simulink model "Circuito"  (R2016b)
settings: Solver=VariableStepAuto  StartTime=0  StopTime=3e-3  RelTol=1e-3
libraries: powerlib x15
settings Model: Creator=Usuario  LastModifiedBy=Usuario
settings DataIOCC: LoggingIntervals=[2e-3, 3e-3]

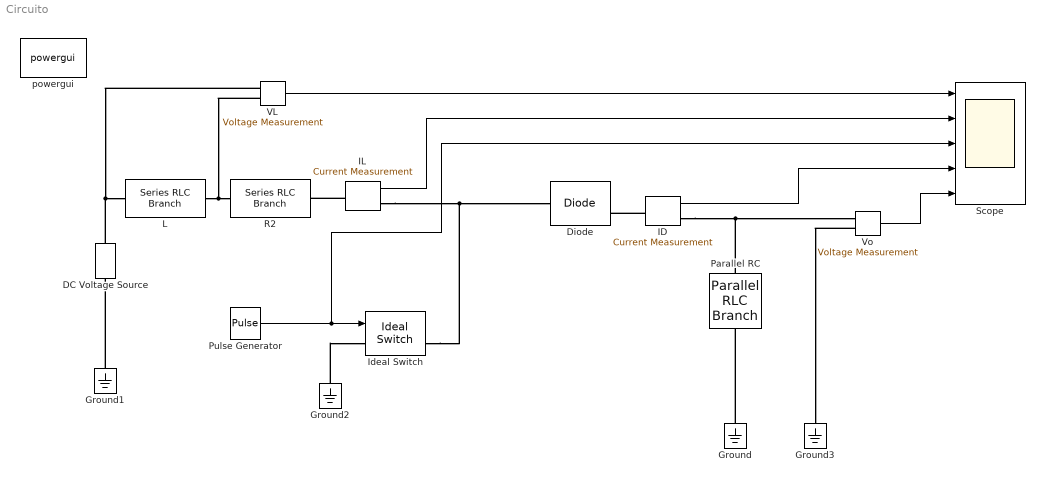
== system Circuito ==
  DC Voltage Source : powerlib/Electrical Sources/DC Voltage Source  Amplitude=12  Measurements=None
  Diode : powerlib/Power Electronics/Diode  Ron=0.001  Lon=0  Vf=0.8  IC=0  UseSnubber=off  Rs=500  Cs=250e-9  Measurements=on
  Ground{,1..3} (4 alike) : powerlib/Elements/Ground  LConnTagsString=a
  ID : powerlib/Measurements/Current Measurement  PhasorSimulation=off  OutputType=Complex  PSBequivalent=0
  IL : powerlib/Measurements/Current Measurement  PhasorSimulation=off  OutputType=Complex  PSBequivalent=0
  Ideal Switch : powerlib/Power Electronics/Ideal Switch  Ron=0.001  Lon=0  IC=0  Rs=1e5  Cs=inf  Measurements=on
  L : powerlib/Elements/Series RLC Branch  LConnTagsString=__new0  RConnTagsString=__new0  BranchType=L  Resistance=1  Inductance=220e-6  SetiL0=off  InitialCurrent=0  Capacitance=1e-6  Setx0=off  InitialVoltage=0  Measurements=None
  Parallel RC : powerlib/Elements/Parallel RLC Branch  LConnTagsString=a  RConnTagsString=__new0  BranchType=RC  Resistance=100  Inductance=0  SetiL0=off  InitialCurrent=0  Capacitance=10e-6  Setx0=off  InitialVoltage=0  Measurements=None
  Pulse Generator : DiscretePulseGenerator  PulseType=Time based  Period=16.667e-6  PulseWidth=54.38447187
  R2 : powerlib/Elements/Series RLC Branch  LConnTagsString=__new0  RConnTagsString=__new0  BranchType=R  Resistance=2  Inductance=1e-3  SetiL0=off  InitialCurrent=0  Capacitance=1e-6  Setx0=off  InitialVoltage=0  Measurements=None
  Scope : Scope  NumInputPorts=5
  VL : powerlib/Measurements/Voltage Measurement  PhasorSimulation=off  OutputType=Complex  PSBequivalent=0
  Vo : powerlib/Measurements/Voltage Measurement  PhasorSimulation=off  OutputType=Complex  PSBequivalent=0
  powergui : powerlib/powergui  Priority=1  SimulationMode=Continuous  SolverType=Tustin/Backward Euler (TBE)  SampleTime=50e-6  frequency=60  SPID=on  DisableSnubberDevices=off  DisableRonSwitches=off  DisableVfSwitches=off  SwTol=0  DisplayEquations=off  Interpol=off  ExternalGateDelay=off  methode=off  Ts=10  FunctionMessages=off  echomessages=off  HookPort=off  EnableUseOfTLC=off  x0status=blocks  frequencyindice=0  Pbase=100e6  ErrMax=1e-4  Iterations=50  UnitsV=kV  UnitsW=MW  buscounter=0  RestoreLinks=warning  ResistiveCurrentMeasurement=off  Frange=[0:2:500]  Ylog=off  Xlog=on  ShowGrid=off  save=off  variable=ZData  structure=0  ZoomFFT=off  StartTime=0.0  cycles=1  DisplayStyle=1  fundamental=60  FreqAxis=off  MaxFrequency=1000  frequencyindicesteady=1  RmsSteady=1  display=off
  wires:
  VL/1 -> Scope/1
  IL/1 -> Scope/2
  Vo/1 -> Scope/5
  ID/1 -> Scope/4
  Pulse Generator/1 -> Ideal Switch/1, Scope/3
  connections:
  Ideal Switch/RConn1 -- IL/RConn1 -- Diode/LConn1
  Parallel RC/LConn1 -- ID/RConn1 -- Vo/LConn1
  Ground/LConn1 -- Parallel RC/RConn1
  Ground1/LConn1 -- DC Voltage Source/LConn1
  Ground2/LConn1 -- Ideal Switch/LConn1
  Vo/LConn2 -- Ground3/LConn1
  IL/LConn1 -- R2/RConn1
  L/RConn1 -- VL/LConn2 -- R2/LConn1
  DC Voltage Source/RConn1 -- VL/LConn1 -- L/LConn1
  ID/LConn1 -- Diode/RConn1
